simulink model "targetingLib"  (R2026b)
settings: Solver=VariableStepAuto
undefined symbols (not defined in the file or in its folder): maxval_sc, minval_sc, modval, samptime, Slope1, Slope2, threshold_add
libraries: hdlsllib x57, simulink x19, simulink_extras x11, dspsigops x2, sl_signal_attributes x2
(part 1 of 3)
settings Model: Creator=The MathWorks, Inc.  LastModifiedBy=vijayenk

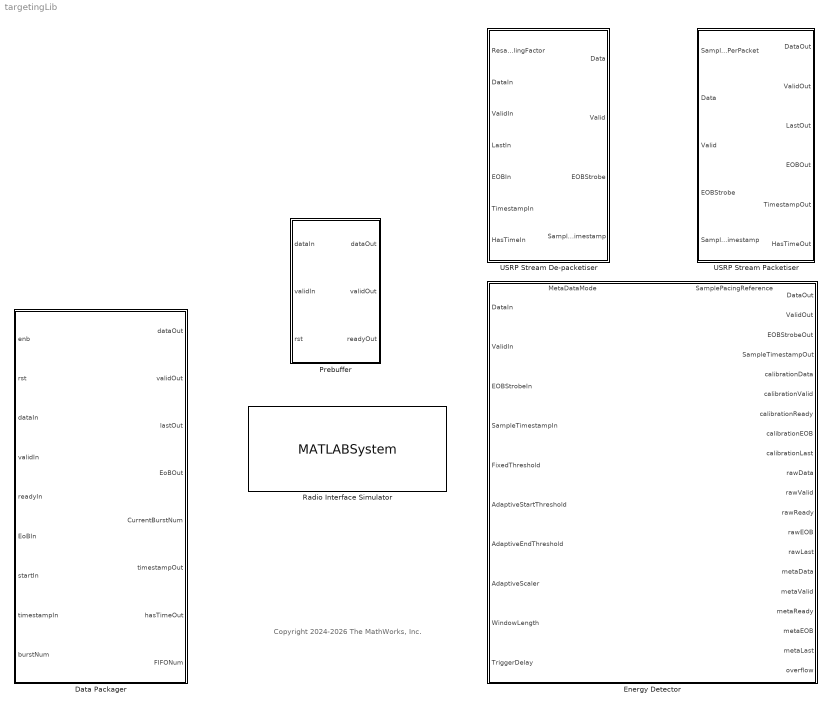
== system targetingLib ==
  note: Copyright 2024-2026 The MathWorks, Inc.
  Data Packager : Subsystem  mask{BufferDepth=12, SPP=256, Mode=Continuous, HasTime=off}
      mask prompts: BufferDepth "Buffer Depth"; HasTime "Use Timestamp"
  Energy Detector : Subsystem
      settings: PortSchema="{\"entries\":[{\"content\":{\"sides\":[{\"content\":{\"connectorIds\":[\"In1\",\"In2\",\"In3\",\"In4\",\"In5\",\"In6\",\"In7\",\"In8\",\"In9\",\"In10\"]},\"type\":\"ConnectorPlacement.EquallySpacedRectSide\",\"uuid\":\"93566f99-0720-4a61-bfb8-f7254dd6d1df\"},{\"content\":{\"connectorIds\":[\"Out1\",\"Out2\",\"Out3\",\"Out4\",\"Out5\",\"Out6\",\"In12\",\"Out7\",\"Out8\",\"Out9\",\"Out10\",\"In13\",\"Out11\",\"Out12\",\"Out13\",\"Out14\",\"In14\",\"Out15\",\"Out16\",\"Out17\"],\"side\":\"RIGHT\"},\"type\":\"ConnectorPlacement.EquallySpacedRectSide\",\"uuid\":\"cdcdfe23-28d5-4579-854c-5ee479bc7078\"},{\"content\":{\"connectorIds\":[\"In11\",\"Out18\"],\"side\":\"TOP\"},\"type\":\"ConnectorPlacement.EquallySpacedRectSide\",\"uuid\":\"28d60382-2d9d-4747-8f66-ca7e1d0bda43\"}]},\"type\":\"ConnectorPlacement.EquallySpacedConnector\",\"uuid\":\"328206bb-f626-4f26-b68f-ea420f212918\"}],\"packageUris\":[\"http://schema.mathworks.com/mf0/Connector/R2020b\"],\"version\":\"1.0\"}"
  Prebuffer : Subsystem  mask{RegisterSize=2048, CyclePerSample=8}
      mask prompts: RegisterSize "Buffer length"; CyclePerSample "Cycle per Sample"
  Radio Interface Simulator : MATLABSystem  System=RadioInterfaceSim  Device=N310  TXRX=TX  ClockSource=Radio  SampleRate=61.44e6  DUTClockRate=61.44e6  InputDataSource=[ 1, 2, 3 ]  ShowOutputStream=off  SimulateUsing=Code generation  ClockUncertainty=off  Uncertainty=0  Jitter=0
      mask Type: RadioInterfaceSim
  USRP Stream De-packetiser : Subsystem
      mask DialogControl DescTextVar Prompt: De-packetiser, convert stream port and sideband signals into data, valid, end of burst strobe and sample timestamp.
      mask Display:
      | disp(...
      |     "USRP Stream" + newline + ...
      |     "De-packetiser" + newline + ...
      |     " " + newline + "Latency: 1")
  USRP Stream Packetiser : Subsystem  mask{MaxSPP=256}
      mask prompts: MaxSPP "Maximum Samples Per Packet:"
      mask DialogControl DescTextVar Prompt: Asserts last signal every SPP number of valids. Delay balances data and valid with last. When EOB_In is asserted with a valid sample both EOB_Out and Last_Out will be asserted and the internal SPP counter is reset.
      mask Display:
      | disp(...
      |     "USRP Stream" + newline + ...
      |     "Packetiser" + newline + ...
      |     " " + newline + "Latency: 1")

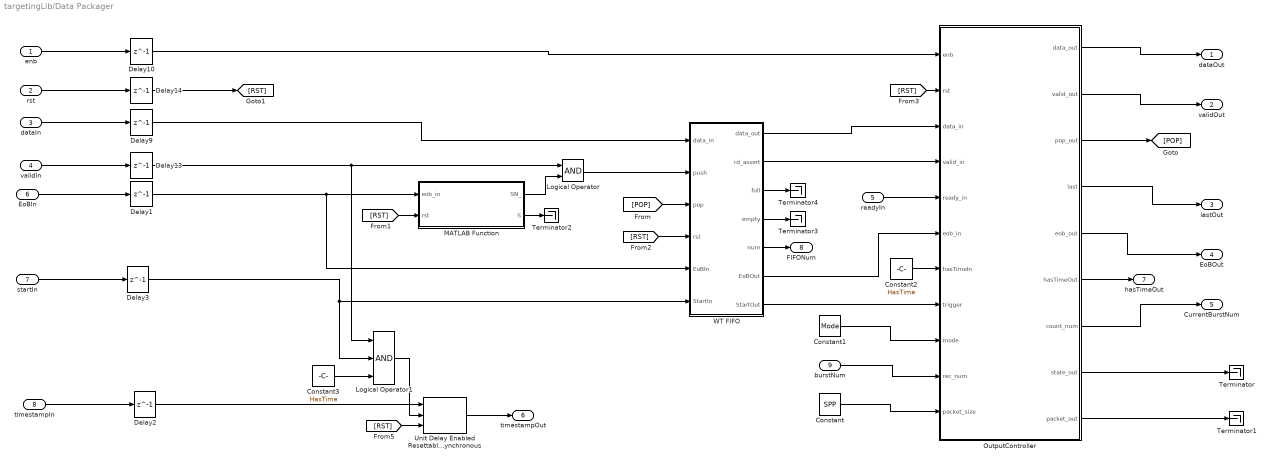
== system targetingLib/Data Packager ==
  enb : Inport
  rst : Inport  Port=2
  dataIn : Inport  Port=3
  validIn : Inport  Port=4
  readyIn : Inport  Port=5
  EoBIn : Inport  Port=6
  startIn : Inport  Port=7
  timestampIn : Inport  Port=8
  burstNum : Inport  Port=9
  Constant : Constant  Value=SPP  OutDataTypeStr=uint16  SampleTime=-1
  Constant1 : Constant  Value=Mode  OutDataTypeStr=boolean  SampleTime=-1
  Constant2 : Constant  Value=HasTime  OutDataTypeStr=boolean  SampleTime=-1
  Constant3 : Constant  Value=HasTime  OutDataTypeStr=boolean  SampleTime=-1
  Delay{1..3,9..10,13..14} (7 alike) : Delay  DelayLength=1  InitialCondition=0
  Logical Operator : Logic  AllPortsSameDT=off  OutDataTypeStr=boolean
  Logical Operator1 : Logic  Inputs=3  AllPortsSameDT=off  OutDataTypeStr=boolean
  MATLAB Function : MATLAB Function  TreatAsAtomicUnit=on
  OutputController : MATLAB Function  TreatAsAtomicUnit=on
  Terminator{,1..4} (5 alike) : Terminator
  Unit Delay Enabled Resettable Synchronous : hdlsllib/Discrete/Unit Delay Enabled Resettable Synchronous  InitialCondition=0.0  SampleTime=-1
  WT FIFO : Subsystem  mask{depth=BufferDepth}
      mask prompts: depth "FIFO Depth"
  dataOut : Outport  VectorParamsAs1DForOutWhenUnconnected=off
  validOut : Outport  Port=2
  lastOut : Outport  Port=3
  EoBOut : Outport  Port=4
  "CurrentBurstNum " : Outport  Port=5
  timestampOut : Outport  Port=6
  hasTimeOut : Outport  Port=7
  FIFONum : Outport  Port=8
  wires:
  readyIn/1 -> OutputController/5(ready_in)
  startIn/1 -> Delay3/1
  Delay3/1 -> Logical Operator1/2, WT FIFO/6(StartIn)
  dataIn/1 -> Delay9/1
  Delay9/1 -> WT FIFO/1(data_in)
  OutputController/5(eob_out) -> EoBOut/1
  OutputController/9(packet_out) -> Terminator1/1
  OutputController/8(state_out) -> Terminator/1
  Delay14/1 -> [RST]
  burstNum/1 -> OutputController/10(rec_num)
  OutputController/7(count_num) -> "CurrentBurstNum "/1
  OutputController/2(valid_out) -> validOut/1
  OutputController/4(last) -> lastOut/1
  validIn/1 -> Delay13/1
  enb/1 -> Delay10/1
  rst/1 -> Delay14/1
  Constant/1 -> OutputController/11(packet_size)
  OutputController/1(data_out) -> dataOut/1
  Delay10/1 -> OutputController/1(enb)
  Logical Operator/1 -> WT FIFO/2(push)
  MATLAB Function/1(SN_) -> Logical Operator/2
  Delay13/1 -> Logical Operator1/1, Logical Operator/1
  WT FIFO/2(rd_assert) -> OutputController/4(valid_in)
  WT FIFO/1(data_out) -> OutputController/3(data_in)
  MATLAB Function/2(S) -> Terminator2/1
  OutputController/3(pop_out) -> [POP]
  [POP] -> WT FIFO/3(pop)
  EoBIn/1 -> Delay1/1
  Delay1/1 -> WT FIFO/5(EoBIn), MATLAB Function/1(eob_in)
  [RST] -> MATLAB Function/2(rst)
  [RST] -> WT FIFO/4(rst)
  [RST] -> OutputController/2(rst)
  Constant1/1 -> OutputController/9(mode)
  timestampIn/1 -> Delay2/1
  [RST] -> Unit Delay Enabled Resettable Synchronous/3
  Delay2/1 -> Unit Delay Enabled Resettable Synchronous/1
  Constant3/1 -> Logical Operator1/3
  Logical Operator1/1 -> Unit Delay Enabled Resettable Synchronous/2
  Unit Delay Enabled Resettable Synchronous/1 -> timestampOut/1
  OutputController/6(hasTimeOut) -> hasTimeOut/1
  WT FIFO/5(num) -> FIFONum/1
  WT FIFO/7(StartOut) -> OutputController/8(trigger)
  WT FIFO/6(EoBOut) -> OutputController/6(eob_in)
  WT FIFO/4(empty) -> Terminator3/1
  WT FIFO/3(full) -> Terminator4/1
  Constant2/1 -> OutputController/7(hasTimeIn)

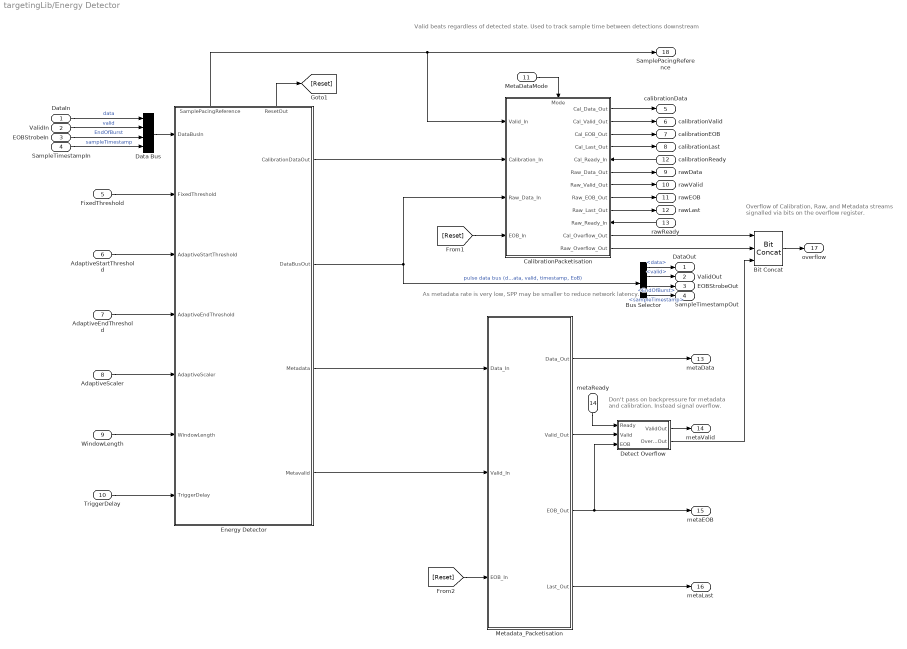
== system targetingLib/Energy Detector ==
  note: Overflow of Calibration, Raw, and Metadata streams signalled via bits on the overflow register.
  note: Don't pass on backpressure for metadata
      |  and calibration. Instead signal overflow.
  note: As metadata rate is very low, SPP may be smaller to reduce network latency.
  note: Valid beats regardless of detected state. Used to track sample time between detections downstream
  DataIn : Inport
  ValidIn : Inport  Port=2
  EOBStrobeIn : Inport  Port=3
  SampleTimestampIn : Inport  Port=4
  FixedThreshold : Inport  Port=5  OutDataTypeStr=single
  AdaptiveStartThreshold : Inport  Port=6  OutDataTypeStr=single
  AdaptiveEndThreshold : Inport  Port=7  OutDataTypeStr=single
  AdaptiveScaler : Inport  Port=8  OutDataTypeStr=single
  WindowLength : Inport  Port=9
  TriggerDelay : Inport  Port=10
  MetaDataMode : Inport  Port=11
  calibrationReady : Inport  Port=12
  rawReady : Inport  Port=13
  metaReady : Inport  Port=14
  Bit Concat : hdlsllib/Logic and Bit Operations/Bit Concat  numInputs=3
  Bus Selector : BusSelector  OutputSignals=data,valid,EndOfBurst,sampleTimestamp
  CalibrationPacketisation : Subsystem
      settings: PortSchema="{\"entries\":[{\"content\":{\"sides\":[{\"content\":{\"connectorIds\":[\"In1\",\"In2\",\"In3\",\"In4\"]},\"type\":\"ConnectorPlacement.EquallySpacedRectSide\",\"uuid\":\"68d3c42e-20fb-4ebf-9d76-09408b5dc78c\"},{\"content\":{\"connectorIds\":[\"Out1\",\"Out2\",\"Out3\",\"Out4\",\"In6\",\"Out5\",\"Out6\",\"Out7\",\"Out8\",\"In7\",\"Out9\",\"Out10\"],\"side\":\"RIGHT\"},\"type\":\"ConnectorPlacement.EquallySpacedRectSide\",\"uuid\":\"04fc1748-9658-4123-a08e-192ddc54cdc2\"},{\"content\":{\"connectorIds\":[\"In5\"],\"side\":\"TOP\"},\"type\":\"ConnectorPlacement.EquallySpacedRectSide\",\"uuid\":\"04b88de6-7de9-43b2-868a-b0760c091651\"}]},\"type\":\"ConnectorPlacement.EquallySpacedConnector\",\"uuid\":\"95b98454-5e5b-460b-bbf7-3c8b216ad478\"}],\"packageUris\":[\"http://schema.mathworks.com/mf0/Connector/R2020b\"],\"version\":\"1.0\"}"
  Data Bus : BusCreator  Inputs=4
  Detect Overflow : Subsystem
  Energy Detector : Subsystem
      settings: PortSchema="{\"entries\":[{\"content\":{\"sides\":[{\"content\":{\"connectorIds\":[\"In1\",\"In2\",\"In3\",\"In4\",\"In5\",\"In6\",\"In7\"]},\"type\":\"ConnectorPlacement.EquallySpacedRectSide\",\"uuid\":\"4ac7fccf-649a-41a5-9bb2-4019e9c8040b\"},{\"content\":{\"connectorIds\":[\"Out1\",\"Out2\",\"Out3\",\"Out4\"],\"side\":\"RIGHT\"},\"type\":\"ConnectorPlacement.EquallySpacedRectSide\",\"uuid\":\"96b2e17e-e1cc-4259-b366-5349f488d48a\"},{\"content\":{\"connectorIds\":[\"Out5\",\"Out6\"],\"side\":\"TOP\"},\"type\":\"ConnectorPlacement.EquallySpacedRectSide\",\"uuid\":\"82faf69d-275a-4a5f-91da-b169cabd35bd\"}]},\"type\":\"ConnectorPlacement.EquallySpacedConnector\",\"uuid\":\"c273b448-1a41-46b6-a8d1-92257bc83a36\"}],\"packageUris\":[\"http://schema.mathworks.com/mf0/Connector/R2020b\"],\"version\":\"1.0\"}"
  Metadata_Packetisation : Subsystem  mask{SPP=3}
      mask prompts: SPP "Samples Per Packet (SPP)"
      mask DialogControl DescGroupVar Prompt: RFNoC Packetisation Handler
      mask DialogControl DescTextVar Prompt: Asserts last signal every SPP number of valids. Delay balances data and valid with last. When EOB_In is asserted with a valid sample both EOB_Out and Last_Out will be asserted and the internal SPP counter is reset.
      mask Display:
      | disp('Packetiser')
      | disp([newline,newline,'Latency: 1'])
  DataOut : Outport
  ValidOut : Outport  Port=2
  EOBStrobeOut : Outport  Port=3
  SampleTimestampOut : Outport  Port=4
  calibrationData : Outport  Port=5
  calibrationValid : Outport  Port=6
  calibrationEOB : Outport  Port=7
  calibrationLast : Outport  Port=8
  rawData : Outport  Port=9
  rawValid : Outport  Port=10
  rawEOB : Outport  Port=11
  rawLast : Outport  Port=12
  metaData : Outport  Port=13
  metaValid : Outport  Port=14
  metaEOB : Outport  Port=15
  metaLast : Outport  Port=16
  overflow : Outport  Port=17
  SamplePacingReference : Outport  Port=18
  wires:
  [Reset] -> CalibrationPacketisation/4(EOB_In)
  CalibrationPacketisation/2(Cal_Valid_Out) -> calibrationValid/1
  CalibrationPacketisation/1(Cal_Data_Out) -> calibrationData/1
  calibrationReady/1 -> CalibrationPacketisation/6(Cal_Ready_In)
  CalibrationPacketisation/8(Raw_Last_Out) -> rawLast/1
  Energy Detector/1(CalibrationDataOut) -> CalibrationPacketisation/2(Calibration_In)
  MetaDataMode/1 -> CalibrationPacketisation/5(Mode)
  CalibrationPacketisation/5(Raw_Data_Out) -> rawData/1
  Metadata_Packetisation/4(Last_Out) -> metaLast/1
  Energy Detector/4(Metavalid) -> Metadata_Packetisation/2(Valid_In)
  WindowLength/1 -> Energy Detector/6(WindowLength)
  rawReady/1 -> CalibrationPacketisation/7(Raw_Ready_In)
  [Reset] -> Metadata_Packetisation/3(EOB_In)
  Energy Detector/6(ResetOut) -> [Reset]
  Energy Detector/5(SamplePacingReference) -> CalibrationPacketisation/1(Valid_In), SamplePacingReference/1
  TriggerDelay/1 -> Energy Detector/7(TriggerDelay)
  FixedThreshold/1 -> Energy Detector/2(FixedThreshold)
  Metadata_Packetisation/3(EOB_Out) -> Detect Overflow/3(EOB), metaEOB/1
  Energy Detector/2(DataBusOut) -> Bus Selector/1, CalibrationPacketisation/3(Raw_Data_In)  "pulse data bus (data, valid, timestamp, EoB)"
  CalibrationPacketisation/4(Cal_Last_Out) -> calibrationLast/1
  CalibrationPacketisation/3(Cal_EOB_Out) -> calibrationEOB/1
  Energy Detector/3(Metadata) -> Metadata_Packetisation/1(Data_In)
  Metadata_Packetisation/1(Data_Out) -> metaData/1
  CalibrationPacketisation/6(Raw_Valid_Out) -> rawValid/1
  AdaptiveScaler/1 -> Energy Detector/5(AdaptiveScaler)
  AdaptiveEndThreshold/1 -> Energy Detector/4(AdaptiveEndThreshold)
  AdaptiveStartThreshold/1 -> Energy Detector/3(AdaptiveStartThreshold)
  CalibrationPacketisation/7(Raw_EOB_Out) -> rawEOB/1
  metaReady/1 -> Detect Overflow/1(Ready)
  Metadata_Packetisation/2(Valid_Out) -> Detect Overflow/2(Valid)
  Detect Overflow/1(ValidOut) -> metaValid/1
  CalibrationPacketisation/10(Raw_Overflow_Out) -> Bit Concat/2
  CalibrationPacketisation/9(Cal_Overflow_Out) -> Bit Concat/1
  Bit Concat/1 -> overflow/1
  Detect Overflow/2(OverflowOut) -> Bit Concat/3
  Data Bus/1 -> Energy Detector/1(DataBusIn)
  DataIn/1 -> Data Bus/1  "data"
  SampleTimestampIn/1 -> Data Bus/4  "sampleTimestamp"
  EOBStrobeIn/1 -> Data Bus/3  "EndOfBurst"
  ValidIn/1 -> Data Bus/2  "valid"
  Bus Selector/1 -> DataOut/1  "<data>"
  Bus Selector/2 -> ValidOut/1  "<valid>"
  Bus Selector/3 -> EOBStrobeOut/1  "<EndOfBurst>"
  Bus Selector/4 -> SampleTimestampOut/1  "<sampleTimestamp>"

== system targetingLib/Prebuffer ==
  dataIn : Inport
  validIn : Inport  Port=2
  rst : Inport  Port=3
  Constant : Constant  Value=floor(RegisterSize/4*3)  OutDataTypeStr=Inherit: Inherit via back propagation  SampleTime=-1
  Constant1 : Constant  Value=floor(RegisterSize/2)  OutDataTypeStr=Inherit: Inherit via back propagation  SampleTime=-1
  Constant2 : Constant  Value=CyclePerSample  OutDataTypeStr=fixdt(0,floor(log2(CyclePerSample))+1,0)  SampleTime=-1
  Delay : Delay  DelayLength=1
  Delay1 : Delay  DelayLength=3
  Delay2 : Delay  DelayLength=1
  HDL FIFO : hdlsllib/HDL RAMs/HDL FIFO  fifo_size=RegisterSize  mode=Classic  ratio=1  dataDim=1  push_msg=Ignore  pop_msg=Ignore  show_empty=on  show_full=on  show_num=on  LabelModeActiveChoice_Mode=Classic  rst_port=on
  Hysteresis Thresholding : Subsystem
  Logical Operator2 : Logic  AllPortsSameDT=off  OutDataTypeStr=boolean
  Terminator : Terminator
  Valid Decimation : Subsystem
  dataOut : Outport
  validOut : Outport  Port=2
  readyOut : Outport  Port=3
  wires:
  dataIn/1 -> HDL FIFO/1
  Delay2/1 -> dataOut/1
  Constant1/1 -> Hysteresis Thresholding/4(LowTh)
  HDL FIFO/4 -> Hysteresis Thresholding/2(CountIn)
  HDL FIFO/1 -> Delay/1
  Delay/1 -> Delay2/1
  Delay1/1 -> validOut/1
  Constant/1 -> Hysteresis Thresholding/3(HighTh)
  validIn/1 -> Logical Operator2/1
  Logical Operator2/1 -> HDL FIFO/2
  rst/1 -> [RST]
  [RST] -> Hysteresis Thresholding/1(rst)
  [RST] -> HDL FIFO/4
  Valid Decimation/1(Pop Out) -> Delay1/1, [POP]
  Constant2/1 -> Valid Decimation/2(ReuseFactor)
  HDL FIFO/2 -> Valid Decimation/3(FIFO Empty)
  [POP] -> HDL FIFO/3
  HDL FIFO/3 -> Terminator/1
  [RST] -> Valid Decimation/1(Rst)
  Hysteresis Thresholding/1(state_out) -> Logical Operator2/2, readyOut/1

== system targetingLib/USRP Stream De-packetiser ==
  ResamplingFactor : Inport  OutDataTypeStr=uint8
  DataIn : Inport  Port=2
  ValidIn : Inport  Port=3
  LastIn : Inport  Port=4
  EOBIn : Inport  Port=5
  TimestampIn : Inport  Port=6
  HasTimeIn : Inport  Port=7
  AND : Logic  IconShape=distinctive  AllPortsSameDT=off  OutDataTypeStr=boolean
  Data Type Conversion : DataTypeConversion  ConvertRealWorld=Stored Integer (SI)  SaturateOnIntegerOverflow=off  RndMeth=Floor
  Delay8 : Delay  DelayLength=1
  Sample Timestamps : Subsystem
  Data : Outport
  Valid : Outport  Port=2
  EOBStrobe : Outport  Port=3
  SampleTimestamp : Outport  Port=4
  wires:
  EOBIn/1 -> AND/2
  LastIn/1 -> AND/1
  AND/1 -> Delay8/1, Sample Timestamps/3(eobStrobeIn)
  Delay8/1 -> Sample Timestamps/4(reset)
  ValidIn/1 -> Sample Timestamps/2(validIn)
  DataIn/1 -> Sample Timestamps/1(dataIn)
  TimestampIn/1 -> Sample Timestamps/5(pktTimestamp)
  HasTimeIn/1 -> Sample Timestamps/6(hasTime)
  Sample Timestamps/1(data) -> Data/1
  Sample Timestamps/2(valid) -> Valid/1
  Sample Timestamps/4(eobStrobe) -> EOBStrobe/1
  Sample Timestamps/3(sampleTimestamp) -> SampleTimestamp/1
  Data Type Conversion/1 -> Sample Timestamps/7(resamplingFactor)
  ResamplingFactor/1 -> Data Type Conversion/1

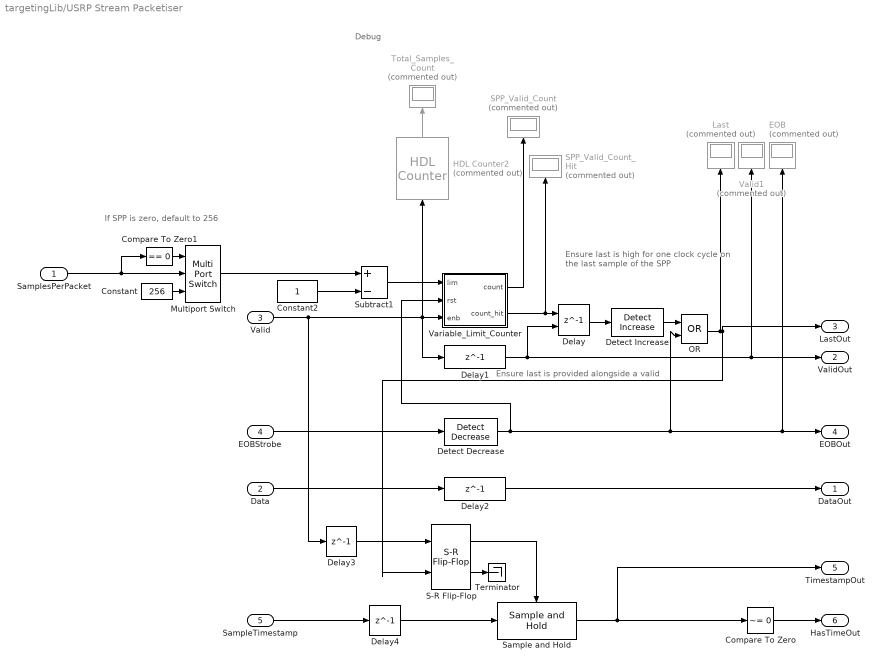
== system targetingLib/USRP Stream Packetiser ==
  note: If SPP is zero, default to 256
  note: Debug
  note: Ensure last is high for one clock cycle
      |  on the last sample of the SPP
  note: Ensure last is provided alongside a valid
  SamplesPerPacket : Inport
  Data : Inport  Port=2
  Valid : Inport  Port=3
  EOBStrobe : Inport  Port=4
  SampleTimestamp : Inport  Port=5
  Compare To Zero : simulink/Logic and Bit Operations/Compare To Zero  relop=~=  OutDataTypeStr=boolean
  Compare To Zero1 : simulink/Logic and Bit Operations/Compare To Zero  relop===  OutDataTypeStr=boolean
  Constant : Constant  Value=256  OutDataTypeStr=Inherit: Inherit via back propagation  SampleTime=-1
  Constant2 : Constant  OutDataTypeStr=fixdt(0,ceil(log2(MaxSPP+1)),0)
  Delay : Delay  DelayLength=1  ShowEnablePort=on
      settings: InputPortMap=u0,e6
  Delay{1..4} (4 alike) : Delay  DelayLength=1
  Detect Decrease : simulink/Logic and Bit Operations/Detect Decrease  vinit=0.0  OutDataTypeStr=boolean
  Detect Increase : simulink/Logic and Bit Operations/Detect Increase  vinit=0.0  OutDataTypeStr=boolean
  EOB : Display  Commented=on
  HDL Counter2 : hdlsllib/Sources/HDL Counter  Commented=on  CountType=Free running  CountInit=0  CountStep=1  CountMax=3  CountFromType=Initial value  CountFrom=0  CountResetPort=off  CountLoadPort=off  CountEnbPort=on  CountDirPort=off  CountHitOutputPort=off  CountDataType=Unsigned  CountWordLen=9  CountFracLen=0  CountSampTime=1
  Last : Display  Commented=on
  Multiport Switch : MultiPortSwitch  DataPortOrder=Zero-based contiguous  Inputs=2  zeroidx=on  OutDataTypeStr=Inherit: Inherit via back propagation  SaturateOnIntegerOverflow=off  InputSameDT=off
  OR : Logic  Operator=OR  IconShape=distinctive  AllPortsSameDT=off  OutDataTypeStr=boolean
  S-R Flip-Flop : simulink_extras/Flip Flops/S-R Flip-Flop  initial_condition=0
  SPP_Valid_Count : Display  Commented=on
  SPP_Valid_Count_Hit : Display  Commented=on
  Sample and Hold : dspsigops/Sample and Hold  trig=Rising edge  initCond=0  latchinput=off
  Subtract1 : Sum  Inputs=+-  OutDataTypeStr=Inherit: Same as first input
  Terminator : Terminator
  Total_Samples_Count : Display  Commented=on
  Valid1 : Display  Commented=on
  Variable_Limit_Counter : Subsystem
  DataOut : Outport
  ValidOut : Outport  Port=2
  LastOut : Outport  Port=3
  EOBOut : Outport  Port=4
  TimestampOut : Outport  Port=5
  HasTimeOut : Outport  Port=6
  wires:
  Constant/1 -> Multiport Switch/3
  Detect Decrease/1 -> Variable_Limit_Counter/2(rst), OR/2, EOBOut/1, EOB/1
  Multiport Switch/1 -> Subtract1/1
  Valid/1 -> Delay3/1, Variable_Limit_Counter/3(enb), HDL Counter2/1, Delay1/1
  Variable_Limit_Counter/2(count_hit) -> Delay/1, SPP_Valid_Count_Hit/1
  HDL Counter2/1 -> Total_Samples_Count/1
  Delay1/1 -> ValidOut/1, Valid1/1, Delay/2
  Detect Increase/1 -> OR/1
  SampleTimestamp/1 -> Delay4/1
  OR/1 -> Last/1, LastOut/1, S-R Flip-Flop/2
  Constant2/1 -> Subtract1/2
  Compare To Zero/1 -> HasTimeOut/1
  SamplesPerPacket/1 -> Compare To Zero1/1, Multiport Switch/2
  Delay/1 -> Detect Increase/1
  Delay3/1 -> S-R Flip-Flop/1
  Variable_Limit_Counter/1(count) -> SPP_Valid_Count/1
  S-R Flip-Flop/2 -> Terminator/1
  Compare To Zero1/1 -> Multiport Switch/1
  Delay2/1 -> DataOut/1
  Sample and Hold/1 -> TimestampOut/1, Compare To Zero/1
  Subtract1/1 -> Variable_Limit_Counter/1(lim)
  Data/1 -> Delay2/1
  EOBStrobe/1 -> Detect Decrease/1
  S-R Flip-Flop/1 -> Sample and Hold/Trigger
  Delay4/1 -> Sample and Hold/1

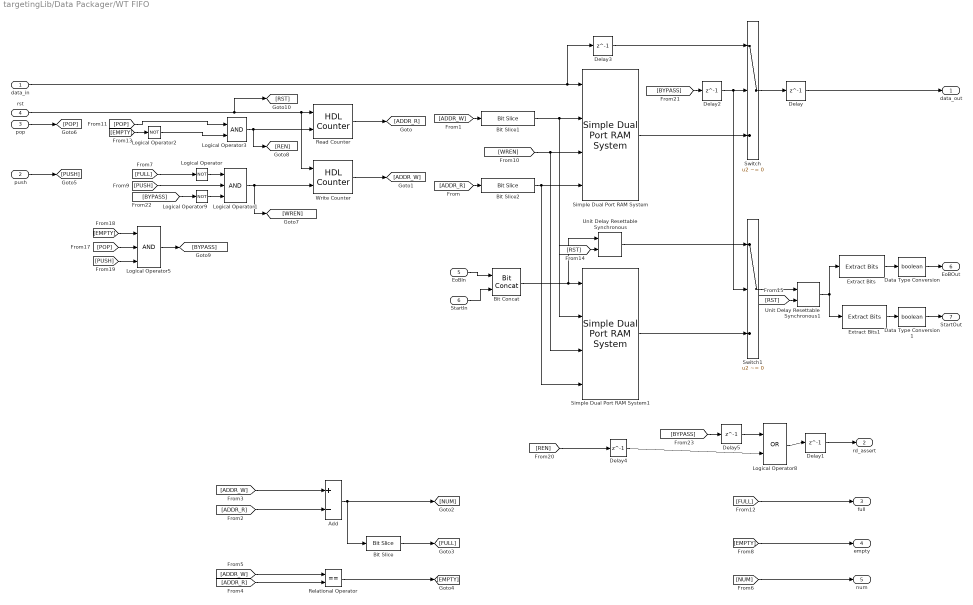
== system targetingLib/Data Packager/WT FIFO ==
  data_in : Inport
  push : Inport  Port=2
  pop : Inport  Port=3
  rst : Inport  Port=4
  EoBIn : Inport  Port=5
  StartIn : Inport  Port=6
  Add : Sum  Inputs=+-  OutDataTypeStr=Inherit: Same as accumulator
  Bit Concat : hdlsllib/Logic and Bit Operations/Bit Concat  numInputs=2
  Bit Slice : hdlsllib/Logic and Bit Operations/Bit Slice  lidx=depth  ridx=depth
  Bit Slice1 : hdlsllib/Logic and Bit Operations/Bit Slice  lidx=depth-1  ridx=0
  Bit Slice2 : hdlsllib/Logic and Bit Operations/Bit Slice  lidx=depth-1  ridx=0
  Data Type Conversion : DataTypeConversion  OutDataTypeStr=boolean  ConvertRealWorld=Stored Integer (SI)  SaturateOnIntegerOverflow=off  RndMeth=Floor
  Data Type Conversion1 : DataTypeConversion  OutDataTypeStr=boolean  ConvertRealWorld=Stored Integer (SI)  SaturateOnIntegerOverflow=off  RndMeth=Floor
  Delay{,1..5} (6 alike) : Delay  DelayLength=1
  Extract Bits : simulink/Logic and Bit Operations/Extract Bits  bitsToExtract=Upper half  numBits=8  bitIdxRange=[0 7]  outScalingMode=Preserve fixed-point scaling
  Extract Bits1 : simulink/Logic and Bit Operations/Extract Bits  bitsToExtract=Lower half  numBits=8  bitIdxRange=[0 7]  outScalingMode=Preserve fixed-point scaling
  Logical Operator : Logic  Operator=NOT  IconShape=distinctive  AllPortsSameDT=off  OutDataTypeStr=boolean
  Logical Operator1 : Logic  Inputs=3  IconShape=distinctive  AllPortsSameDT=off  OutDataTypeStr=boolean
  Logical Operator2 : Logic  Operator=NOT  IconShape=distinctive  AllPortsSameDT=off  OutDataTypeStr=boolean
  Logical Operator3 : Logic  IconShape=distinctive  AllPortsSameDT=off  OutDataTypeStr=boolean
  Logical Operator5 : Logic  Inputs=3  IconShape=distinctive  AllPortsSameDT=off  OutDataTypeStr=boolean
  Logical Operator8 : Logic  Operator=OR  IconShape=distinctive  AllPortsSameDT=off  OutDataTypeStr=boolean
  Logical Operator9 : Logic  Operator=NOT  IconShape=distinctive  AllPortsSameDT=off  OutDataTypeStr=boolean
  Read Counter : hdlsllib/Sources/HDL Counter  CountType=Free running  CountInit=0  CountStep=1  CountMax=25  CountFromType=Initial value  CountFrom=0  CountResetPort=on  CountLoadPort=off  CountEnbPort=on  CountDirPort=off  CountHitOutputPort=off  CountDataType=Unsigned  CountWordLen=depth+1  CountFracLen=0  CountSampTime=1
  Relational Operator : RelationalOperator  Operator===  OutDataTypeStr=boolean  RndMeth=Simplest  InputSameDT=off
  Simple Dual Port RAM System : hdlsllib/HDL RAMs/Simple Dual Port RAM System  RAMType=Simple dual port  AsyncRead=off  WriteOutputValue=New data  RAMInitialValue=0  allowBusInputs=off  WritesHaveOutput=on  NumReads=0  NumWrites=1  SimulateUsing=Code generation  ModelRAMDelay=on  VectorAccess=Parallel
  Simple Dual Port RAM System1 : hdlsllib/HDL RAMs/Simple Dual Port RAM System  RAMType=Simple dual port  AsyncRead=off  WriteOutputValue=New data  RAMInitialValue=0  allowBusInputs=off  WritesHaveOutput=on  NumReads=0  NumWrites=1  SimulateUsing=Code generation  ModelRAMDelay=on  VectorAccess=Parallel
  Switch : Switch  Criteria=u2 ~= 0  SaturateOnIntegerOverflow=off  InputSameDT=off
  Switch1 : Switch  Criteria=u2 ~= 0  SaturateOnIntegerOverflow=off  InputSameDT=off
  Unit Delay Resettable Synchronous : hdlsllib/Discrete/Unit Delay Resettable Synchronous  InitialCondition=0.0  SampleTime=-1
  Unit Delay Resettable Synchronous1 : hdlsllib/Discrete/Unit Delay Resettable Synchronous  InitialCondition=0.0  SampleTime=-1
  Write Counter : hdlsllib/Sources/HDL Counter  CountType=Free running  CountInit=0  CountStep=1  CountMax=25  CountFromType=Initial value  CountFrom=0  CountResetPort=on  CountLoadPort=off  CountEnbPort=on  CountDirPort=off  CountHitOutputPort=off  CountDataType=Unsigned  CountWordLen=depth+1  CountFracLen=0  CountSampTime=1
  data_out : Outport
  rd_assert : Outport  Port=2
  full : Outport  Port=3
  empty : Outport  Port=4
  num : Outport  Port=5
  EoBOut : Outport  Port=6
  StartOut : Outport  Port=7
  wires:
  pop/1 -> [POP]
  [EMPTY] -> empty/1
  Logical Operator1/1 -> Write Counter/2, [WREN]
  [ADDR_W] -> Add/1
  Logical Operator/1 -> Logical Operator1/1
  [PUSH] -> Logical Operator1/2
  [ADDR_R] -> Add/2
  [FULL] -> full/1
  Read Counter/1 -> [ADDR_R]
  Bit Slice/1 -> [FULL]
  data_in/1 -> Delay3/1, Simple Dual Port RAM System/1
  [FULL] -> Logical Operator/1
  [ADDR_W] -> Bit Slice1/1
  Write Counter/1 -> [ADDR_W]
  Relational Operator/1 -> [EMPTY]
  [NUM] -> num/1
  [ADDR_R] -> Bit Slice2/1
  Bit Slice1/1 -> Simple Dual Port RAM System1/2, Simple Dual Port RAM System/2
  Bit Slice2/1 -> Simple Dual Port RAM System1/4, Simple Dual Port RAM System/4
  Logical Operator3/1 -> Read Counter/2, [REN]
  [POP] -> Logical Operator3/1
  [EMPTY] -> Logical Operator2/1
  Logical Operator2/1 -> Logical Operator3/2
  Add/1 -> [NUM], Bit Slice/1
  [ADDR_R] -> Relational Operator/2
  [ADDR_W] -> Relational Operator/1
  [WREN] -> Simple Dual Port RAM System1/3, Simple Dual Port RAM System/3
  [BYPASS] -> Delay2/1
  Switch/1 -> Delay/1
  Delay/1 -> data_out/1
  [PUSH] -> Logical Operator5/3
  [POP] -> Logical Operator5/2
  [EMPTY] -> Logical Operator5/1
  Logical Operator8/1 -> Delay1/1
  Delay1/1 -> rd_assert/1
  Simple Dual Port RAM System/1 -> Switch/3
  Delay2/1 -> Switch/2, Switch1/2
  Logical Operator9/1 -> Logical Operator1/3
  Delay3/1 -> Switch/1
  Logical Operator5/1 -> [BYPASS]
  [BYPASS] -> Logical Operator9/1
  [REN] -> Delay4/1
  [BYPASS] -> Delay5/1
  Delay4/1 -> Logical Operator8/2
  Delay5/1 -> Logical Operator8/1
  rst/1 -> [RST], Write Counter/1, Read Counter/1
  push/1 -> [PUSH]
  Switch1/1 -> Unit Delay Resettable Synchronous1/1
  Simple Dual Port RAM System1/1 -> Switch1/3
  Unit Delay Resettable Synchronous/1 -> Switch1/1
  Bit Concat/1 -> Unit Delay Resettable Synchronous/1, Simple Dual Port RAM System1/1
  EoBIn/1 -> Bit Concat/1
  StartIn/1 -> Bit Concat/2
  Extract Bits/1 -> Data Type Conversion/1
  Extract Bits1/1 -> Data Type Conversion1/1
  Unit Delay Resettable Synchronous1/1 -> Extract Bits/1, Extract Bits1/1
  [RST] -> Unit Delay Resettable Synchronous/2
  [RST] -> Unit Delay Resettable Synchronous1/2
  Data Type Conversion/1 -> EoBOut/1
  Data Type Conversion1/1 -> StartOut/1

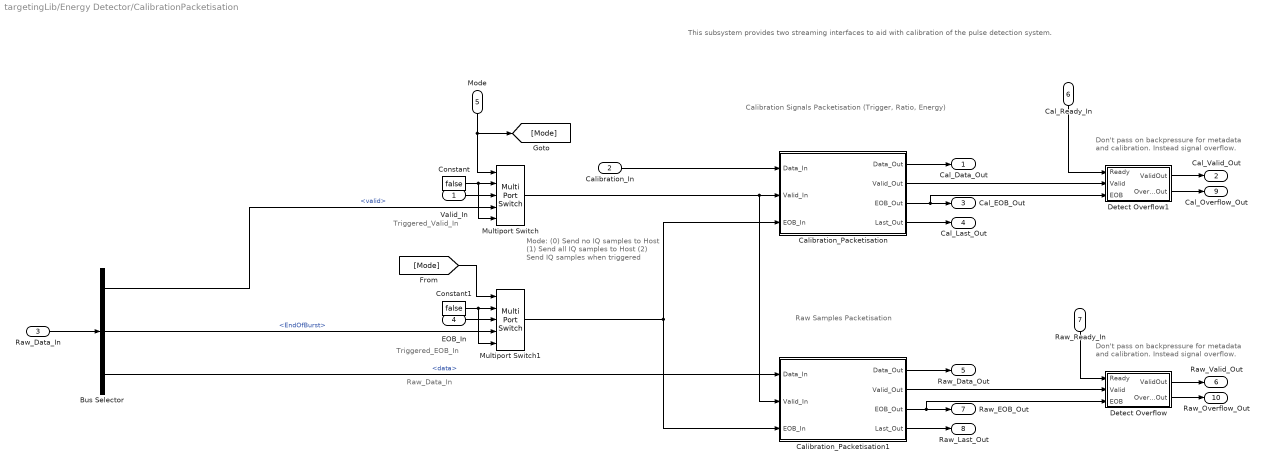
== system targetingLib/Energy Detector/CalibrationPacketisation ==
  note: Raw_Data_In
  note: Triggered_EOB_In
  note: Triggered_Valid_In
  note: Mode:
      | (0) Send no IQ samples to Host
      | (1) Send all IQ samples to Host
      | (2) Send IQ samples when triggered
  note: This subsystem provides two streaming interfaces to aid with calibration of the pulse detection system.
  note: Raw Samples Packetisation
  note: Calibration Signals Packetisation (Trigger, Ratio, Energy)
  note: Don't pass on backpressure for metadata
      |  and calibration. Instead signal overflow.
  note: Don't pass on backpressure for metadata
      |  and calibration. Instead signal overflow.
  Valid_In : Inport
  Calibration_In : Inport  Port=2
  Raw_Data_In : Inport  Port=3
  EOB_In : Inport  Port=4
  Mode : Inport  Port=5
  Cal_Ready_In : Inport  Port=6
  Raw_Ready_In : Inport  Port=7
  Bus Selector : BusSelector  OutputSignals=valid,EndOfBurst,data
  Calibration_Packetisation : Subsystem  mask{SPP=1024}
      mask prompts: SPP "Samples Per Packet (SPP)"
      mask DialogControl DescGroupVar Prompt: RFNoC Packetisation Handler
      mask DialogControl DescTextVar Prompt: Asserts last signal every SPP number of valids. Delay balances data and valid with last. When EOB_In is asserted with a valid sample both EOB_Out and Last_Out will be asserted and the internal SPP counter is reset.
      mask Display:
      | disp('Packetiser')
      | disp([newline,newline,'Latency: 1'])
  Calibration_Packetisation1 : Subsystem  mask{SPP=1024}
      mask prompts: SPP "Samples Per Packet (SPP)"
      mask DialogControl DescGroupVar Prompt: RFNoC Packetisation Handler
      mask DialogControl DescTextVar Prompt: Asserts last signal every SPP number of valids. Delay balances data and valid with last. When EOB_In is asserted with a valid sample both EOB_Out and Last_Out will be asserted and the internal SPP counter is reset.
      mask Display:
      | disp('Packetiser')
      | disp([newline,newline,'Latency: 1'])
  Constant : Constant  Value=false
  Constant1 : Constant  Value=false
  Detect Overflow : Subsystem
  Detect Overflow1 : Subsystem
  Multiport Switch : MultiPortSwitch  DataPortOrder=Zero-based contiguous  DataPortForDefault=Additional data port  zeroidx=on  OutDataTypeStr=Inherit: Keep MSB  SaturateOnIntegerOverflow=off  InputSameDT=off
  Multiport Switch1 : MultiPortSwitch  DataPortOrder=Zero-based contiguous  DataPortForDefault=Additional data port  zeroidx=on  OutDataTypeStr=Inherit: Keep MSB  SaturateOnIntegerOverflow=off  InputSameDT=off
  Cal_Data_Out : Outport
  Cal_Valid_Out : Outport  Port=2
  Cal_EOB_Out : Outport  Port=3
  Cal_Last_Out : Outport  Port=4
  Raw_Data_Out : Outport  Port=5
  Raw_Valid_Out : Outport  Port=6
  Raw_EOB_Out : Outport  Port=7
  Raw_Last_Out : Outport  Port=8
  Cal_Overflow_Out : Outport  Port=9
  Raw_Overflow_Out : Outport  Port=10
  wires:
  Calibration_Packetisation/3(EOB_Out) -> Cal_EOB_Out/1, Detect Overflow1/3(EOB)
  Calibration_Packetisation/2(Valid_Out) -> Detect Overflow1/2(Valid)
  Calibration_Packetisation/4(Last_Out) -> Cal_Last_Out/1
  Multiport Switch1/1 -> Calibration_Packetisation1/3(EOB_In), Calibration_Packetisation/3(EOB_In)
  Detect Overflow1/1(ValidOut) -> Cal_Valid_Out/1
  Calibration_Packetisation/1(Data_Out) -> Cal_Data_Out/1
  Multiport Switch/1 -> Calibration_Packetisation1/2(Valid_In), Calibration_Packetisation/2(Valid_In)
  Detect Overflow/1(ValidOut) -> Raw_Valid_Out/1
  Calibration_In/1 -> Calibration_Packetisation/1(Data_In)
  Cal_Ready_In/1 -> Detect Overflow1/1(Ready)
  Calibration_Packetisation1/3(EOB_Out) -> Detect Overflow/3(EOB), Raw_EOB_Out/1
  Calibration_Packetisation1/4(Last_Out) -> Raw_Last_Out/1
  Calibration_Packetisation1/1(Data_Out) -> Raw_Data_Out/1
  Calibration_Packetisation1/2(Valid_Out) -> Detect Overflow/2(Valid)
  Bus Selector/3 -> Calibration_Packetisation1/1(Data_In)  "<data>"
  Raw_Ready_In/1 -> Detect Overflow/1(Ready)
  Mode/1 -> Multiport Switch/1, [Mode]
  Valid_In/1 -> Multiport Switch/3
  Bus Selector/1 -> Multiport Switch/4  "<valid>"
  Constant/1 -> Multiport Switch/5, Multiport Switch/2
  Bus Selector/2 -> Multiport Switch1/4  "<EndOfBurst>"
  [Mode] -> Multiport Switch1/1
  EOB_In/1 -> Multiport Switch1/3
  Constant1/1 -> Multiport Switch1/5, Multiport Switch1/2
  Raw_Data_In/1 -> Bus Selector/1
  Detect Overflow1/2(OverflowOut) -> Cal_Overflow_Out/1
  Detect Overflow/2(OverflowOut) -> Raw_Overflow_Out/1

== system targetingLib/Energy Detector/Detect Overflow ==
  note: Throw away if not ready.
      | Assume will always be ready due to low rates.
  Ready : Inport
  Valid : Inport  Port=2
  EOB : Inport  Port=3
  AND1 : Logic  IconShape=distinctive  AllPortsSameDT=off  OutDataTypeStr=boolean
  AND2 : Logic  IconShape=distinctive  AllPortsSameDT=off  OutDataTypeStr=boolean
  Delay : Delay  DelayLength=1
  NOT : Logic  Operator=NOT  IconShape=distinctive  AllPortsSameDT=off  OutDataTypeStr=boolean
  Reset on next burst : simulink_extras/Flip Flops/S-R Flip-Flop  initial_condition=0
  Start of Burst : Subsystem
  Terminator : Terminator
  ValidOut : Outport
  OverflowOut : Outport  Port=2
  wires:
  AND1/1 -> ValidOut/1
  Ready/1 -> AND1/2, NOT/1
  Valid/1 -> AND2/2, Start of Burst/1(Valid), AND1/1  "Valid"
  NOT/1 -> AND2/1
  EOB/1 -> Start of Burst/2(EOB)  "EOB"
  Start of Burst/1(SOB) -> Reset on next burst/2
  AND2/1 -> Delay/1
  Reset on next burst/1 -> OverflowOut/1
  Reset on next burst/2 -> Terminator/1
  Delay/1 -> Reset on next burst/1

== system targetingLib/Energy Detector/Energy Detector ==
  note: Optionally delay trigger by up to
      | 63 samples to account for window size
  note: Use the sample pacing reference to keep internal DUT time synchronised with data arriving from the radio in cases where the DUT clock rate does not match the baseband sample rate.
  DataBusIn : Inport
  FixedThreshold : Inport  Port=2
  AdaptiveStartThreshold : Inport  Port=3
  AdaptiveEndThreshold : Inport  Port=4
  AdaptiveScaler : Inport  Port=5
  WindowLength : Inport  Port=6
  TriggerDelay : Inport  Port=7
  Bus Selector : BusSelector  OutputSignals=valid
  Create Meta Data Stream : Subsystem
  Delay : Delay  DelayLengthSource=Input port  DelayLengthUpperLimit=63  ShowEnablePort=on
      settings: InputPortMap=u0,p1,e6
  Delay1 : Delay
  Delay3 : Delay
  Energy Detector : Subsystem
      settings: PortSchema="{\"entries\":[{\"content\":{\"sides\":[{\"content\":{\"connectorIds\":[\"In1\"]},\"type\":\"ConnectorPlacement.EquallySpacedRectSide\",\"uuid\":\"0de094d3-167a-4085-94fc-e8417bfd92d8\"},{\"content\":{\"connectorIds\":[\"Out1\",\"Out2\",\"Out3\",\"Out4\"],\"side\":\"RIGHT\"},\"type\":\"ConnectorPlacement.EquallySpacedRectSide\",\"uuid\":\"33ebd278-bafd-4c71-ad90-d3dcfa3515b5\"},{\"content\":{\"connectorIds\":[\"In2\",\"In3\",\"In4\",\"In5\",\"In6\"],\"side\":\"TOP\"},\"type\":\"ConnectorPlacement.EquallySpacedRectSide\",\"uuid\":\"e2754c58-db2d-48cd-bf1d-3435700e27b8\"}]},\"type\":\"ConnectorPlacement.EquallySpacedConnector\",\"uuid\":\"3abe9e58-cf74-4122-ac44-ba13f783cb21\"}],\"packageUris\":[\"http://schema.mathworks.com/mf0/Connector/R2020b\"],\"version\":\"1.0\"}"
  Triggered Burst Formatting : Subsystem
  CalibrationDataOut : Outport
  DataBusOut : Outport  Port=2
  Metadata : Outport  Port=3
  Metavalid : Outport  Port=4
  SamplePacingReference : Outport  Port=5
  ResetOut : Outport  Port=6
  wires:
  DataBusIn/1 -> Energy Detector/1(DataBusIn)
  AdaptiveStartThreshold/1 -> Energy Detector/3(AdaptiveThreshold)
  AdaptiveScaler/1 -> Energy Detector/5(AdaptiveThresholdScaler)
  FixedThreshold/1 -> Energy Detector/6(FixedThreshold)
  Energy Detector/3(Triggered) -> Delay/1  "ED_Trigger"
  Energy Detector/2(DataBusOut) -> Bus Selector/1, Triggered Burst Formatting/1(Data_Bus_In)  "ED_DataOut"
  Triggered Burst Formatting/1(Data_Bus_Out) -> Create Meta Data Stream/2(Triggered_Data_Bus_Out), DataBusOut/1  "ED_Data_Bus_Out"
  Delay1/1 -> SamplePacingReference/1
  AdaptiveEndThreshold/1 -> Energy Detector/4(AdaptiveEndThreshold)
  Delay/1 -> Triggered Burst Formatting/2(Trigger)  "ED_Trigger_Delay"
  WindowLength/1 -> Energy Detector/2(WindowLength)
  TriggerDelay/1 -> Delay/2
  Delay3/1 -> CalibrationDataOut/1
  Energy Detector/4(CalibrationOut) -> Delay3/1
  Triggered Burst Formatting/2(Reset_Out) -> ResetOut/1  "ED_Reset_Out"
  Bus Selector/1 -> Delay1/1, Delay/3  "<valid>"
  Energy Detector/1(Energy) -> Create Meta Data Stream/1(Energy)
  Create Meta Data Stream/1(Meta_Data_Data) -> Metadata/1
  Create Meta Data Stream/2(Meta_Data_Valid) -> Metavalid/1

== system targetingLib/Energy Detector/Metadata_Packetisation ==
  note: Debug
  note: Ensure last is provided alongside a valid
  note: Ensure last is high for one clock cycle
      |  on the last sample of the SPP
  Data_In : Inport
  Valid_In : Inport  Port=2
  EOB_In : Inport  Port=3
  Delay : Delay  DelayLength=1  ShowEnablePort=on
      settings: InputPortMap=u0,e6
  Delay1 : Delay  DelayLength=1
  Delay2 : Delay  DelayLength=1
  Detect Decrease : simulink/Logic and Bit Operations/Detect Decrease  vinit=0.0  OutDataTypeStr=boolean
  Detect Increase : simulink/Logic and Bit Operations/Detect Increase  vinit=0.0  OutDataTypeStr=boolean
  EOB : Display  Commented=on
  HDL Counter1 : hdlsllib/Sources/HDL Counter  CountType=Count limited  CountInit=0  CountStep=1  CountMax=SPP-1  CountFromType=Initial value  CountFrom=0  CountResetPort=on  CountLoadPort=off  CountEnbPort=on  CountDirPort=off  CountHitOutputPort=on  CountDataType=Unsigned  CountWordLen=ceil(log2(SPP))  CountFracLen=0  CountSampTime=1
  HDL Counter2 : hdlsllib/Sources/HDL Counter  Commented=on  CountType=Free running  CountInit=0  CountStep=1  CountMax=3  CountFromType=Initial value  CountFrom=0  CountResetPort=off  CountLoadPort=off  CountEnbPort=on  CountDirPort=off  CountHitOutputPort=off  CountDataType=Unsigned  CountWordLen=9  CountFracLen=0  CountSampTime=1
  Last : Display  Commented=on
  OR : Logic  Operator=OR  IconShape=distinctive  AllPortsSameDT=off  OutDataTypeStr=boolean
  SPP_Valid_Count : Display  Commented=on
  SPP_Valid_Count_Hit : Display  Commented=on
  Total_Samples_Count : Display  Commented=on
  Valid : Display  Commented=on
  Data_Out : Outport
  Valid_Out : Outport  Port=2
  EOB_Out : Outport  Port=3
  Last_Out : Outport  Port=4
  wires:
  Delay2/1 -> Data_Out/1
  Delay1/1 -> Valid_Out/1, Valid/1, Delay/2
  Valid_In/1 -> HDL Counter1/2, Delay1/1, HDL Counter2/1
  HDL Counter2/1 -> Total_Samples_Count/1
  HDL Counter1/2 -> Delay/1, SPP_Valid_Count_Hit/1
  Data_In/1 -> Delay2/1
  HDL Counter1/1 -> SPP_Valid_Count/1
  EOB_In/1 -> Detect Decrease/1
  Delay/1 -> Detect Increase/1
  Detect Increase/1 -> OR/1
  OR/1 -> Last/1, Last_Out/1
  Detect Decrease/1 -> HDL Counter1/1, OR/2, EOB_Out/1, EOB/1

== system targetingLib/Prebuffer/Hysteresis Thresholding ==
  rst : Inport
  CountIn : Inport  Port=2
  HighTh : Inport  Port=3
  LowTh : Inport  Port=4
  Delay1 : Delay  DelayLength=1  InitialCondition=0
  Delay2 : Delay  DelayLength=1  InitialCondition=0
  Delay20 : Delay  DelayLength=1  InitialCondition=0
  Hysteresis Th : MATLAB Function  TreatAsAtomicUnit=on
  Logical Operator : Logic  Operator=NOT  IconShape=distinctive  AllPortsSameDT=off  OutDataTypeStr=boolean
  Relational Operator : RelationalOperator  Operator=>  OutDataTypeStr=boolean  RndMeth=Simplest  InputSameDT=off
  Relational Operator2 : RelationalOperator  Operator=<  OutDataTypeStr=boolean  RndMeth=Simplest  InputSameDT=off
  state_out : Outport
  wires:
  Relational Operator2/1 -> Delay20/1
  Relational Operator/1 -> Delay1/1
  CountIn/1 -> Relational Operator2/1, Relational Operator/1
  Hysteresis Th/1(state_out) -> Logical Operator/1
  LowTh/1 -> Relational Operator2/2
  HighTh/1 -> Relational Operator/2
  rst/1 -> Delay2/1
  Delay20/1 -> Hysteresis Th/3(th_L)
  Delay1/1 -> Hysteresis Th/2(th_H)
  Delay2/1 -> Hysteresis Th/1(rst)
  Logical Operator/1 -> state_out/1

== system targetingLib/Prebuffer/Valid Decimation ==
  Rst : Inport
  ReuseFactor : Inport  Port=2
  FIFO Empty : Inport  Port=3
  HDL Counter : hdlsllib/Sources/HDL Counter  CountType=Free running  CountInit=1  CountStep=1  CountMax=25  CountFromType=Initial value  CountFrom=1  CountResetPort=on  CountLoadPort=off  CountEnbPort=on  CountDirPort=off  CountHitOutputPort=off  CountDataType=Unsigned  CountWordLen=floor(log2(CyclePerSample))+1  CountFracLen=0  CountSampTime=1
  Logical Operator : Logic  Operator=NOT  AllPortsSameDT=off  OutDataTypeStr=boolean
  Logical Operator1 : Logic  Operator=OR  AllPortsSameDT=off  OutDataTypeStr=boolean
  Logical Operator3 : Logic  AllPortsSameDT=off  OutDataTypeStr=boolean
  Relational Operator : RelationalOperator  Operator===  OutDataTypeStr=boolean  RndMeth=Simplest  InputSameDT=off
  Pop Out : Outport
  wires:
  Logical Operator/1 -> HDL Counter/2, Logical Operator3/2
  ReuseFactor/1 -> Relational Operator/1
  Relational Operator/1 -> Logical Operator1/1, Logical Operator3/1
  Logical Operator1/1 -> HDL Counter/1
  HDL Counter/1 -> Relational Operator/2
  FIFO Empty/1 -> Logical Operator/1
  Rst/1 -> Logical Operator1/2
  Logical Operator3/1 -> Pop Out/1

== system targetingLib/USRP Stream De-packetiser/Sample Timestamps ==
  note: Loading introduced 1 cycle delay since we use the start of a valid packet as loader signal
  dataIn : Inport
  validIn : Inport  Port=2
  eobStrobeIn : Inport  Port=3
  reset : Inport  Port=4
  pktTimestamp : Inport  Port=5
  hasTime : Inport  Port=6
  resamplingFactor : Inport  Port=7  OutDataTypeStr=uint64
  AND1 : Logic  IconShape=distinctive  AllPortsSameDT=off  OutDataTypeStr=boolean
  Delay1 : Delay  DelayLength=1
  Delay2 : Delay  DelayLength=1
  Delay3 : Delay  DelayLength=1
  Detect Increase2 : simulink/Logic and Bit Operations/Detect Increase  vinit=0.0  OutDataTypeStr=boolean
  Packet timestamp 2 Sample timestamp : Subsystem  mask(HDL Counter){CountType=Free running, CountInit=0, CountStep=1, CountMax=25, CountFromType=Initial value, CountFrom=0, CountResetPort=on, CountLoadPort=on, CountEnbPort=on, CountDirPort=off, CountHitOutputPort=off, CountDataType=Unsigned, CountWordLen=64, CountFracLen=0, CountSampTime=1}
      mask prompts: CountType "Simulink:masks:CounterType_MP"; CountInit "Simulink:masks:InitialValue_MP"; CountStep "Simulink:masks:StepValue_MP"; CountMax "Simulink:masks:CountToValue_MP"; CountFromType "Simulink:masks:CountFrom_MP"; CountFrom "Simulink:masks:CountFromValue_MP"; CountResetPort "Simulink:masks:LocalReset_MP"; CountLoadPort "Simulink:masks:LoadPorts_MP"; CountEnbPort "Simulink:masks:CountEnable_MP"; CountDirPort "Simulink:masks:CountDirection_MP"; CountHitOutputPort "Simulink:masks:CountHit_MP"; CountDataType "Simulink:masks:CountOutputData_MP"; CountWordLen "Simulink:masks:WordLength_MP"; CountFracLen "Simulink:masks:FractionLength_MP"; CountSampTime "Simulink:masks:SampleTime_MP"
      mask help: Simulink:masks:HDLCounter_MD
      mask init:
      | issigned = double(strcmp(get_param(gcb, 'CountDataType'), 'Signed'));
      | [maxval_sc,freerun,  samptime, threshold_add, modval,  minval_sc, modulo] = hdlblkmask_counter;
      mask Help: helpview([docroot '/hdlcoder/helptargets.map'],'HDL_Counter');
      mask TypeOptions CountType: Free running | Count limited | Modulo
      mask Callback CountType: hdlblkmask_counter
      mask Callback CountInit: hdlblkmask_counter
      mask TypeOptions CountFromType: Initial value | Specify
      mask Callback CountFromType: hdlblkmask_counter
      mask Callback CountResetPort: hdlblkmask_counter
      mask Callback CountLoadPort: hdlblkmask_counter
      mask Callback CountEnbPort: hdlblkmask_counter
      mask Callback CountDirPort: hdlblkmask_counter
      mask Callback CountHitOutputPort: hdlblkmask_counter
      mask TypeOptions CountDataType: Unsigned | Signed
      mask DialogControl CountType Prompt: Counter type:
      mask DialogControl CountInit Prompt: Initial value:
      mask DialogControl CountStep Prompt: Step value:
      mask DialogControl CountMax Prompt: Count to value:
      mask DialogControl CountFromType Prompt: Count from:
      mask DialogControl CountFrom Prompt: Count from value:
      mask DialogControl CountResetPort Prompt: Local reset port
      mask DialogControl CountLoadPort Prompt: Load ports
      mask DialogControl CountEnbPort Prompt: Count enable port
      mask DialogControl CountDirPort Prompt: Count direction port
      mask DialogControl CountHitOutputPort Prompt: Count hit output port
      mask DialogControl CountDataType Prompt: Counter output data is:
      mask DialogControl CountWordLen Prompt: Word length:
      mask DialogControl CountFracLen Prompt: Fraction length:
      mask DialogControl CountSampTime Prompt: Sample time:
  data : Outport
  valid : Outport  Port=2
  sampleTimestamp : Outport  Port=3
  eobStrobe : Outport  Port=4
  wires:
  Packet timestamp 2 Sample timestamp/1(count) -> sampleTimestamp/1  "sampleTimestamp"
  reset/1 -> Packet timestamp 2 Sample timestamp/1(rst)
  dataIn/1 -> Delay2/1
  validIn/1 -> Packet timestamp 2 Sample timestamp/4(enb), Delay1/1
  pktTimestamp/1 -> Packet timestamp 2 Sample timestamp/3(load_val), Detect Increase2/1
  Delay1/1 -> valid/1  "valid"
  eobStrobeIn/1 -> Delay3/1
  Delay3/1 -> eobStrobe/1  "EndOfBurst"
  hasTime/1 -> AND1/1
  AND1/1 -> Packet timestamp 2 Sample timestamp/2(load)
  Detect Increase2/1 -> AND1/2
  Delay2/1 -> data/1  "data"
  resamplingFactor/1 -> Packet timestamp 2 Sample timestamp/5(step)

== system targetingLib/USRP Stream Packetiser/Variable_Limit_Counter ==
  lim : Inport
  rst : Inport  Port=2
  enb : Inport  Port=3
  Delay : Delay  DelayLength=1  InitialCondition=1
  Equal : RelationalOperator  OutDataTypeStr=boolean  RndMeth=Simplest  InputSameDT=off
  HDL Counter : hdlsllib/Sources/HDL Counter  CountType=Free running  CountInit=0  CountStep=1  CountMax=25  CountFromType=Initial value  CountFrom=0  CountResetPort=on  CountLoadPort=off  CountEnbPort=on  CountDirPort=off  CountHitOutputPort=off  CountDataType=Unsigned  CountWordLen=ceil(log2(MaxSPP+1))  CountFracLen=0  CountSampTime=1
  OR1 : Logic  Operator=OR  IconShape=distinctive  AllPortsSameDT=off  OutDataTypeStr=boolean
  count : Outport
  count_hit : Outport  Port=2
  wires:
  enb/1 -> HDL Counter/2
  lim/1 -> Delay/1
  Equal/1 -> OR1/2, count_hit/1
  OR1/1 -> HDL Counter/1
  HDL Counter/1 -> count/1, Equal/1
  rst/1 -> OR1/1
  Delay/1 -> Equal/2

== system targetingLib/Energy Detector/CalibrationPacketisation/Calibration_Packetisation ==
  note: Debug
  note: Ensure last is provided alongside a valid
  note: Ensure last is high for one clock cycle
      |  on the last sample of the SPP
  Data_In : Inport
  Valid_In : Inport  Port=2
  EOB_In : Inport  Port=3
  Delay : Delay  DelayLength=1  ShowEnablePort=on
      settings: InputPortMap=u0,e6
  Delay1 : Delay  DelayLength=1
  Delay2 : Delay  DelayLength=1
  Detect Decrease : simulink/Logic and Bit Operations/Detect Decrease  vinit=0.0  OutDataTypeStr=boolean
  Detect Increase : simulink/Logic and Bit Operations/Detect Increase  vinit=0.0  OutDataTypeStr=boolean
  EOB : Display  Commented=on
  HDL Counter1 : hdlsllib/Sources/HDL Counter  CountType=Count limited  CountInit=0  CountStep=1  CountMax=SPP-1  CountFromType=Initial value  CountFrom=0  CountResetPort=on  CountLoadPort=off  CountEnbPort=on  CountDirPort=off  CountHitOutputPort=on  CountDataType=Unsigned  CountWordLen=ceil(log2(SPP))  CountFracLen=0  CountSampTime=1
  HDL Counter2 : hdlsllib/Sources/HDL Counter  Commented=on  CountType=Free running  CountInit=0  CountStep=1  CountMax=3  CountFromType=Initial value  CountFrom=0  CountResetPort=off  CountLoadPort=off  CountEnbPort=on  CountDirPort=off  CountHitOutputPort=off  CountDataType=Unsigned  CountWordLen=9  CountFracLen=0  CountSampTime=1
  Last : Display  Commented=on
  OR : Logic  Operator=OR  IconShape=distinctive  AllPortsSameDT=off  OutDataTypeStr=boolean
  SPP_Valid_Count : Display  Commented=on
  SPP_Valid_Count_Hit : Display  Commented=on
  Total_Samples_Count : Display  Commented=on
  Valid : Display  Commented=on
  Data_Out : Outport
  Valid_Out : Outport  Port=2
  EOB_Out : Outport  Port=3
  Last_Out : Outport  Port=4
  wires:
  Delay2/1 -> Data_Out/1
  Delay1/1 -> Valid_Out/1, Valid/1, Delay/2
  Valid_In/1 -> HDL Counter1/2, Delay1/1, HDL Counter2/1
  HDL Counter2/1 -> Total_Samples_Count/1
  HDL Counter1/2 -> Delay/1, SPP_Valid_Count_Hit/1
  Data_In/1 -> Delay2/1
  HDL Counter1/1 -> SPP_Valid_Count/1
  EOB_In/1 -> Detect Decrease/1
  Delay/1 -> Detect Increase/1
  Detect Increase/1 -> OR/1
  OR/1 -> Last/1, Last_Out/1
  Detect Decrease/1 -> HDL Counter1/1, OR/2, EOB_Out/1, EOB/1

== system targetingLib/Energy Detector/CalibrationPacketisation/Calibration_Packetisation1 ==
  note: Debug
  note: Ensure last is provided alongside a valid
  note: Ensure last is high for one clock cycle
      |  on the last sample of the SPP
  Data_In : Inport
  Valid_In : Inport  Port=2
  EOB_In : Inport  Port=3
  Delay : Delay  DelayLength=1  ShowEnablePort=on
      settings: InputPortMap=u0,e6
  Delay1 : Delay  DelayLength=1
  Delay2 : Delay  DelayLength=1
  Detect Decrease : simulink/Logic and Bit Operations/Detect Decrease  vinit=0.0  OutDataTypeStr=boolean
  Detect Increase : simulink/Logic and Bit Operations/Detect Increase  vinit=0.0  OutDataTypeStr=boolean
  EOB : Display  Commented=on
  HDL Counter1 : hdlsllib/Sources/HDL Counter  CountType=Count limited  CountInit=0  CountStep=1  CountMax=SPP-1  CountFromType=Initial value  CountFrom=0  CountResetPort=on  CountLoadPort=off  CountEnbPort=on  CountDirPort=off  CountHitOutputPort=on  CountDataType=Unsigned  CountWordLen=ceil(log2(SPP))  CountFracLen=0  CountSampTime=1
  HDL Counter2 : hdlsllib/Sources/HDL Counter  Commented=on  CountType=Free running  CountInit=0  CountStep=1  CountMax=3  CountFromType=Initial value  CountFrom=0  CountResetPort=off  CountLoadPort=off  CountEnbPort=on  CountDirPort=off  CountHitOutputPort=off  CountDataType=Unsigned  CountWordLen=9  CountFracLen=0  CountSampTime=1
  Last : Display  Commented=on
  OR : Logic  Operator=OR  IconShape=distinctive  AllPortsSameDT=off  OutDataTypeStr=boolean
  SPP_Valid_Count : Display  Commented=on
  SPP_Valid_Count_Hit : Display  Commented=on
  Total_Samples_Count : Display  Commented=on
  Valid : Display  Commented=on
  Data_Out : Outport
  Valid_Out : Outport  Port=2
  EOB_Out : Outport  Port=3
  Last_Out : Outport  Port=4
  wires:
  Delay2/1 -> Data_Out/1
  Delay1/1 -> Valid_Out/1, Valid/1, Delay/2
  Valid_In/1 -> HDL Counter1/2, Delay1/1, HDL Counter2/1
  HDL Counter2/1 -> Total_Samples_Count/1
  HDL Counter1/2 -> Delay/1, SPP_Valid_Count_Hit/1
  Data_In/1 -> Delay2/1
  HDL Counter1/1 -> SPP_Valid_Count/1
  EOB_In/1 -> Detect Decrease/1
  Delay/1 -> Detect Increase/1
  Detect Increase/1 -> OR/1
  OR/1 -> Last/1, Last_Out/1
  Detect Decrease/1 -> HDL Counter1/1, OR/2, EOB_Out/1, EOB/1

== system targetingLib/Energy Detector/CalibrationPacketisation/Detect Overflow ==
  note: Throw away if not ready.
      | Assume will always be ready due to low rates.
  Ready : Inport
  Valid : Inport  Port=2
  EOB : Inport  Port=3
  AND1 : Logic  IconShape=distinctive  AllPortsSameDT=off  OutDataTypeStr=boolean
  AND2 : Logic  IconShape=distinctive  AllPortsSameDT=off  OutDataTypeStr=boolean
  Delay : Delay  DelayLength=1
  NOT : Logic  Operator=NOT  IconShape=distinctive  AllPortsSameDT=off  OutDataTypeStr=boolean
  Reset on next burst : simulink_extras/Flip Flops/S-R Flip-Flop  initial_condition=0
  Start of Burst : Subsystem
  Terminator : Terminator
  ValidOut : Outport
  OverflowOut : Outport  Port=2
  wires:
  AND1/1 -> ValidOut/1
  Ready/1 -> AND1/2, NOT/1
  Valid/1 -> AND2/2, Start of Burst/1(Valid), AND1/1  "Valid"
  NOT/1 -> AND2/1
  EOB/1 -> Start of Burst/2(EOB)  "EOB"
  Start of Burst/1(SOB) -> Reset on next burst/2
  AND2/1 -> Delay/1
  Reset on next burst/1 -> OverflowOut/1
  Reset on next burst/2 -> Terminator/1
  Delay/1 -> Reset on next burst/1
